simulink library "SolarCollector"  (R2018b)
settings: Solver=ode45  StartTime=0.0  StopTime=10.0  RelTol=1e-3  EnableMultiTasking=on
undefined symbols (not defined in the file): path_carnot
libraries: carnot x5
settings Model: Creator=bernd.hafner  LastModifiedBy=drhf
settings DataIOCC: LimitDataPoints=on  SaveFormat=Array  SignalLoggingSaveFormat=ModelDataLogs
settings OptimizationCC: ExpressionDepthLimit=2147483647  LifeSpan=inf
settings DebuggingCC: UnderspecifiedInitializationDetection=Classic  MergeDetectMultiDrivingBlocksExec=none  SolverPrmCheckMsg=warning  FcnCallInpInsideContextMsg=warning  StateNameClashWarn=warning  SFUnexpectedBacktrackingDiag=warning  SFNoUnconditionalDefaultTransitionDiag=warning  SFExecutionAtInitializationDiag=none
settings HardwareCC: ProdBitPerPointer=32  ProdBitPerSizeT=32  ProdBitPerPtrDiffT=32  ProdLargestAtomicFloat=None  ProdIntDivRoundTo=Undefined  ProdEndianess=Unspecified  ProdWordSize=32  ProdHWDeviceType=32-bit Generic
settings ModelReferenceCC: PropagateSignalLabelsOutOfModel=off
settings SFSimCC: SimUseLocalCustomCode=off
settings RTWCC: RTWUseLocalCustomCode=off
settings CodeAppCC: StateflowObjectComments=on
settings GRTTargetCC: TargetLangStandard=C89/C90 (ANSI)  GeneratePreprocessorConditionals=Disable all  CombineOutputUpdateFcns=off  GRTInterface=on
settings ConfigComp: CovMetricSettings=dw  CovHtmlReporting=on  CovSaveCumulativeToWorkspaceVar=on  CovSaveSingleToWorkspaceVar=on  CovExternalEMLEnable=off

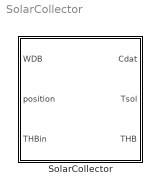
== system SolarCollector ==
  SolarCollector : Subsystem  mask(Solar Thermal Collector){t0=20, Ncollector=1, PathName=fullfile(path_carnot('libsl'), 'Source', 'Solar_Thermal', 'SolarCollector', 'parameter_set'), FileName='DefaultCollector.mat', userPath=off, userParam=off, acol=3.5, len=0.1, fta=0.7, c1=1.1, c2=0.001, c3=0, c4=0, c5=5000, c6=0, KbAngles=[0 5 10 15 20 25 30 35 40 45 50 55 60 65 70 75 80 85 90], KbL=[1 1 0.9999 0.9996 0.9991 0.9982 0.9965 0.9935 0.9886 0.9807 0.9678 0.9473 0.9148 0.8638 0.7846 0.6644 0.4907 0.2599 0], KbT=[1 1 1 1 1 1 1 1 1 1 1 0.875 0.75 0.625 0.5 0.375 0.25 0.125 0], Kd=0.92, dplin=10, dpqua=10, SensorTimeConstant=10}
      mask prompts: t0 "Initial temperature [°C]"; Ncollector "Number of collectors in parallel"; PathName "Path"; FileName "Parameter set"; userPath "Edit path and name of parameter set"; userParam "User defined parameters"; acol "A: surface  of one collector module in m²"; len "Length between collector inlet and outlet in m"; fta "Fin Efficiency * Transmission * Absorption (F'(tau alfa))"; c1 "c1 : heat loss coefficient at (Tm-Ta)=0  [W/(m²*K)]"; c2 "c2: temperature dependence of the heat loss coefficient [W/(m*K)²]"; c3 "c3 : wind speed dependence of the heat loss coefficient [J/(m³K)]"; c4 "c4 : sky temperature dependence of the heat loss coefficient [W/(m²K)]"; c5 "c5 : effective thermal capacity [J/(m²K)]"; c6 "c6 : wind dependence in the zero loss efficiency [s/m]"; KbAngles "Kb: angles for longitudinal and transversal IAM [degree]"; KbL "KbL: values for longitudinal incidence angle modifier (0..1)"; KbT "KbT: values for transversal incidence angle modifier (0..1)"; Kd "Kd : Incidence angle modifier diffuse radiation"; dplin "lin: linear pressure drop in Pa/(kg/s)"; dpqua "qua: quadratic pressure drop in Pa/(kg/s)²"; SensorTimeConstant "time constant of sensor [s]"
      mask help:
      | Model for glazed solar thermal collector according to ISO 9806 standard.
      | c5 dTm/dt = F'(TauAlfa) (Kdir Idir + Kdfu Idfu) - (Tm-Tamb) (c1 + c2 (Tm-Tamb)) - v_wind (c3 (Tm-Ta) + c6 Iglb) + c4 (ELongwave - sigma_SB Tamb^4) - mdot cp (Tout-Tin) /A
      | Tm = (Tin+Tout)/2
      | Keep in mind that the ISO equation is not respecting the energy conservation for variable inlet conditions (e.g. temperature).
      | IT IS RECOMMENDED TO USE THIS MODEL ONLY FOR STEADY STATE CONDITIONS AT THE INLET (use Collector_Unglazed_ISO_2node model for system simulation).
      mask init:
      | % callback to set parameters of model
      | [ok, param] = CarnotCallbacks_CollectorEN12975Conf('SetParameters',gcbh,PathName,FileName);
      mask Help: web(fullfile(path_carnot('help'),'collector_en12975.html'),'-helpbrowser')
      mask TypeOptions t0: T_Sensor/t0 | glazed_collector_ISO9806/tini
      mask TypeOptions Ncollector: Ncollector/Value | Gain1/Gain | Gain2/Gain
      mask Callback userPath: [ok, param] = CarnotCallbacks_CollectorEN12975Conf('UserEdit',gcbh);
      mask Callback userParam: [ok, param] = CarnotCallbacks_CollectorEN12975Conf('UserEdit',gcbh);
      mask TypeOptions acol: glazed_collector_ISO9806/acol | Acol/Value
      mask TypeOptions len: Pressure_Drop_Collector/len
      mask TypeOptions fta: glazed_collector_ISO9806/fta
      mask TypeOptions c1: glazed_collector_ISO9806/c1
      mask TypeOptions c2: glazed_collector_ISO9806/c2
      mask TypeOptions c3: glazed_collector_ISO9806/c3
      mask TypeOptions c4: glazed_collector_ISO9806/c4
      mask TypeOptions c5: glazed_collector_ISO9806/c5
      mask TypeOptions c6: glazed_collector_ISO9806/c6
      mask TypeOptions KbAngles: glazed_collector_ISO9806/kblangle | glazed_collector_ISO9806/kbtangle
      mask TypeOptions KbL: glazed_collector_ISO9806/KbL
      mask TypeOptions KbT: glazed_collector_ISO9806/KbT
      mask TypeOptions Kd: glazed_collector_ISO9806/Kd
      mask TypeOptions dplin: Pressure_Drop_Collector/lin
      mask TypeOptions dpqua: Pressure_Drop_Collector/qua
      mask TypeOptions SensorTimeConstant: T_Sensor/tc
      mask DialogControl ParameterGroupVar Prompt: Picking a parameter set
      mask DialogControl Control2 Prompt: Carnot public data
      mask DialogControl Control2 Callback: [ok, file] = CarnotCallbacks_CollectorEN12975Conf('GetFilename',gcbh,'public');
      mask DialogControl Control3 Prompt: Carnot internal data
      mask DialogControl Control3 Callback: [ok, file] = CarnotCallbacks_CollectorEN12975Conf('GetFilename',gcbh,'internal');
      mask DialogControl Control4 Prompt: Selected path
      mask DialogControl Control4 Callback: [ok, file] = CarnotCallbacks_CollectorEN12975Conf('GetFilename',gcbh,'selected');
      mask DialogControl Container7 Prompt: Geometry
      mask DialogControl Container8 Prompt: Coll.Params
      mask DialogControl Container9 Prompt: Optics
      mask DialogControl Container10 Prompt: Hydraulic
      mask DialogControl Container11 Prompt: Sensors
      mask DialogControl Control5 Prompt: Save in Carnot interal data
      mask DialogControl Control5 Callback: [ok, param] = CarnotCallbacks_CollectorEN12975Conf('SaveFilename',gcbh,'internal','COL');
      mask DialogControl Control6 Prompt: Save in seleced path
      mask DialogControl Control6 Callback: [ok, param] = CarnotCallbacks_CollectorEN12975Conf('SaveFilename',gcbh,'selected','COL');
      mask Display:
      | % user defined picture file
      | picfile = fullfile(path_carnot('intlibsl'), ...
      |     'Source','Solar_Thermal','SolarCollector','parameter_set', ...
      |      'Collector_CONF.jpg');
      | 
      | pic = false;
      | 
      | % show internal picture if defined
      | if ~BlockIsInCarnotLibrary    % if not located in library any more
      |     if exist(picfile)
      |         image(imread(picfile), [0.2, 0, 0.6, 1])
      |         set_param(gcb, 'BackgroundColor', 'White')
      |         pic = true;
      |     end
      | end
      | 
      | if ~pic    % show public picture
      |     disp('Solar Thermal\nCollector\n\nISO 9806')
      |     set_param(gcb, 'BackgroundColor', 'Yellow')
      | end

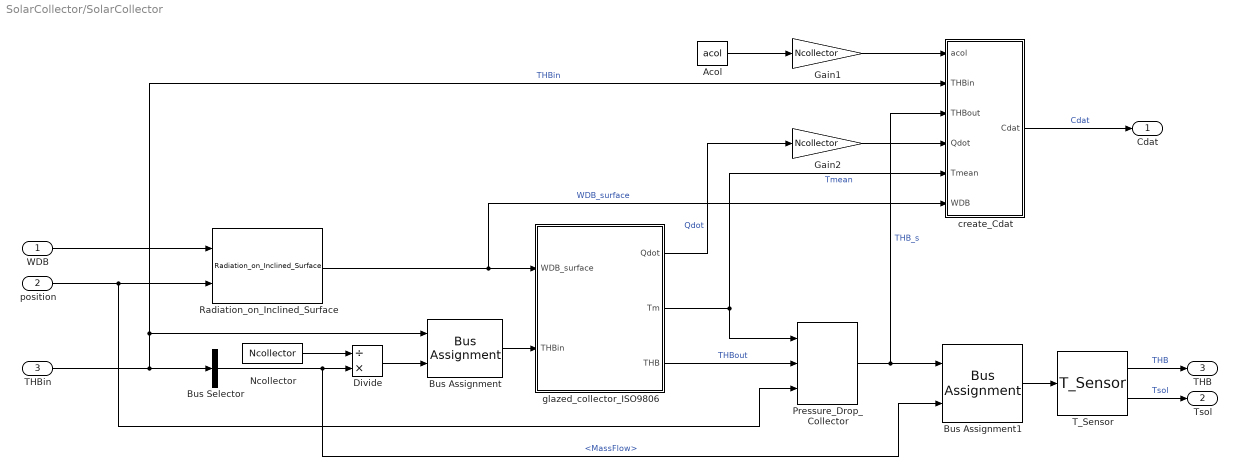
== system SolarCollector/SolarCollector ==
  WDB : Inport
  position : Inport  Port=2
  THBin : Inport  Port=3
  Acol : Constant  Value=acol
  Bus Assignment : BusAssignment  AssignedSignals=MassFlow
  Bus Assignment1 : BusAssignment  AssignedSignals=MassFlow
  Bus Selector : BusSelector  OutputSignals=MassFlow
  Divide : Product  Inputs=/*
  Gain1 : Gain  Gain=Ncollector
  Gain2 : Gain  Gain=Ncollector
  Ncollector : Constant  Value=Ncollector
  Pressure_Drop_Collector : carnot/Basic/Pressure_Drop/Pressure_Drop_Collector  len=len  lin=dplin  qua=dpqua
      settings: SourceProductName=Carnot
  Radiation_on_Inclined_Surface : carnot/Weather/Radiation_on_Inclined_Surface  sky=Perez 1990  reflect=0.2
      settings: SourceProductName=Carnot
  T_Sensor : carnot/Control/T_Sensor  tc=SensorTimeConstant  t0=t0
      settings: SourceProductName=Carnot
  create_Cdat : Subsystem
  glazed_collector_ISO9806 : Subsystem  mask(Basic Solar Thermal Collector){acol=acol, fta=fta, c1=c1, c2=c2, c3=c3, c4=c4, c5=c5, c6=c6, tini=t0, kblangle=KbAngles, KbL=KbL, kbtangle=KbAngles, KbT=KbT, Kd=Kd}
      mask prompts: acol "A : collector surface  [m²]"; fta "Fin Efficiency * Transmission * Absorption (F'(tau alfa))"; c1 "c1 : heat loss coefficient at (Tm-Ta)=0  [W/(m²*K)]"; c2 "c2: temperature dependence of the heat loss coefficient [W/(m*K)²]"; c3 "c3 : wind speed dependence of the heat loss coefficient [J/(m³K)]"; c4 "c4 : sky temperature dependence of the heat loss coefficient [W/(m²K)]"; c5 "c5 : effective thermal capacity [J/(m²K)]"; c6 "c6 : wind dependence in the zero loss efficiency [s/m]"; tini "initial temperature [degree Celsius]"; kblangle "KbL: angles for longitudinal IAM [degree]"; KbL "KbL: values for longitudinal incidence angle modifier (0..1)"; kbtangle "KbT: angles for transversal IAM [degree]"; KbT "KbT: values for transversal incidence angle modifier (0..1)"; Kd "Kd : Incidence angle modifier diffuse radiation"
      mask help: Model according to EN 12975 / ISO 22975
      mask Help: web(fullfile(path_carnot('help'),'Solar_Collector_basic.html'),'-helpbrowser')
      mask TypeOptions fta: IAM_Table_KbL_KbT/fta
      mask TypeOptions kblangle: IAM_Table_KbL_KbT/kblangle
      mask TypeOptions KbL: IAM_Table_KbL_KbT/KbL
      mask TypeOptions kbtangle: IAM_Table_KbL_KbT/kbtangle
      mask TypeOptions KbT: IAM_Table_KbL_KbT/KbT
      mask TypeOptions Kd: IAM_Table_KbL_KbT/Kd
      mask DialogControl Container4 Prompt: Collector Parameters
      mask DialogControl Container10 Prompt: Optics
      mask Display: disp('glazed\nsolar\nthermal\ncollector\nISO 9806')
  Cdat : Outport
  Tsol : Outport  Port=2
  THB : Outport  Port=3
  wires:
  Bus Assignment/1 -> glazed_collector_ISO9806/2(THBin)
  T_Sensor/1 -> THB/1  "THB"
  T_Sensor/2 -> Tsol/1  "Tsol"
  Divide/1 -> Bus Assignment/2
  Ncollector/1 -> Divide/1
  WDB/1 -> Radiation_on_Inclined_Surface/1
  glazed_collector_ISO9806/1(Qdot) -> Gain2/1  "Qdot"
  glazed_collector_ISO9806/3(THB) -> Pressure_Drop_Collector/2  "THBout"
  THBin/1 -> Bus Selector/1, create_Cdat/2(THBin), Bus Assignment/1  "THBin"
  glazed_collector_ISO9806/2(Tm) -> Pressure_Drop_Collector/1, create_Cdat/5(Tmean)  "Tmean"
  create_Cdat/1(Cdat) -> Cdat/1  "Cdat"
  Radiation_on_Inclined_Surface/1 -> glazed_collector_ISO9806/1(WDB_surface), create_Cdat/6(WDB)  "WDB_surface"
  Pressure_Drop_Collector/1 -> create_Cdat/3(THBout), Bus Assignment1/1  "THB_s"
  position/1 -> Pressure_Drop_Collector/3, Radiation_on_Inclined_Surface/2
  Acol/1 -> Gain1/1
  Bus Selector/1 -> Bus Assignment1/2, Divide/2  "<MassFlow>"
  Gain1/1 -> create_Cdat/1(acol)
  Gain2/1 -> create_Cdat/4(Qdot)
  Bus Assignment1/1 -> T_Sensor/1

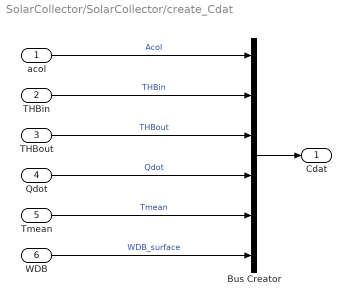
== system SolarCollector/SolarCollector/create_Cdat ==
  acol : Inport
  THBin : Inport  Port=2
  THBout : Inport  Port=3
  Qdot : Inport  Port=4
  Tmean : Inport  Port=5
  WDB : Inport  Port=6
  Bus Creator : BusCreator  Inputs=6
  Cdat : Outport
  wires:
  Tmean/1 -> Bus Creator/5  "Tmean"
  Qdot/1 -> Bus Creator/4  "Qdot"
  Bus Creator/1 -> Cdat/1
  WDB/1 -> Bus Creator/6  "WDB_surface"
  THBout/1 -> Bus Creator/3  "THBout"
  THBin/1 -> Bus Creator/2  "THBin"
  acol/1 -> Bus Creator/1  "Acol"

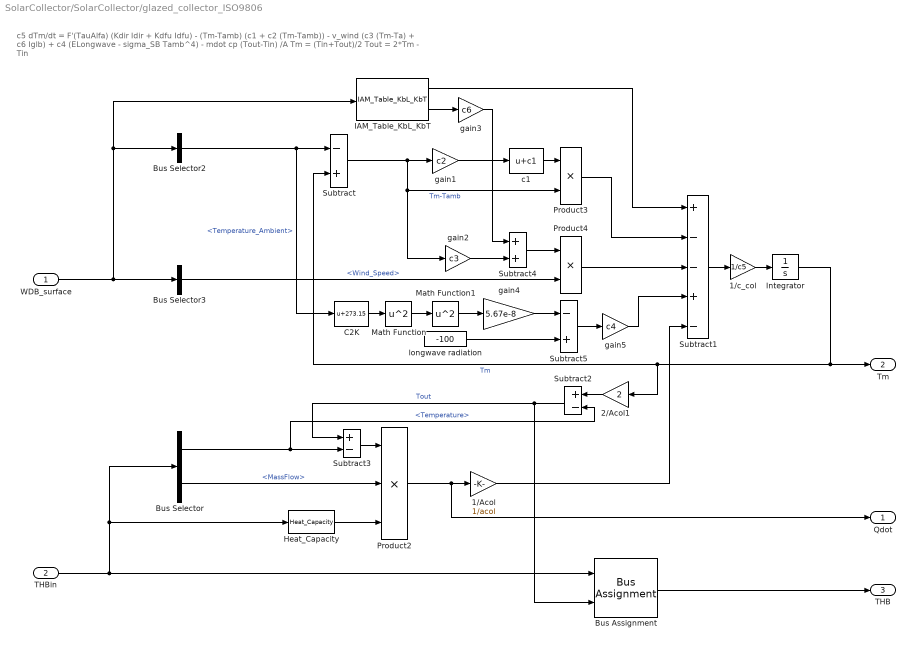
== system SolarCollector/SolarCollector/glazed_collector_ISO9806 ==
  note: c5 dTm/dt = F'(TauAlfa) (Kdir Idir + Kdfu Idfu) - (Tm-Tamb) (c1 + c2 (Tm-Tamb)) - v_wind (c3 (Tm-Ta) + c6 Iglb) + c4 (ELongwave - sigma_SB Tamb^4) - mdot cp (Tout-Tin) /A
      | Tm = (Tin+Tout)/2
      | Tout = 2*Tm - Tin
  WDB_surface : Inport
  THBin : Inport  Port=2
  1/Acol : Gain  Gain=1/acol
  1/c_col : Gain  Gain=1/c5
  2/Acol1 : Gain  Gain=2
  Bus Assignment : BusAssignment  AssignedSignals=Temperature
  Bus Selector : BusSelector  OutputSignals=Temperature,MassFlow
  Bus Selector2 : BusSelector  OutputSignals=Temperature_Ambient
  Bus Selector3 : BusSelector  OutputSignals=Wind_Speed
  C2K : Bias  Bias=273.15
  Heat_Capacity : carnot/Basic/Material_Properties/Heat_Capacity  VariantControl=CarlibClassic  INPUTARGUMENTS=THB  DEBUGLEVEL=DEBUGLEVEL  MAXTOTALWARNINGS=inf  MAXCONSECUTIVEWARNINGS=inf  WRITETOFILE=0  FILENAME='errors.txt'
      settings: SourceProductName=Carnot
  IAM_Table_KbL_KbT : carnot/Source/Solar_Thermal/IncidenceAngleModifier/IAM_Table_KbL_KbT  fta=fta  kblangle=kblangle  KbL=KbL  kbtangle=kbtangle  KbT=KbT  Kd=Kd
      settings: SourceProductName=Carnot
  Integrator : Integrator  InitialCondition=tini
  Math Function : Math  Operator=square  SaturateOnIntegerOverflow=on
  Math Function1 : Math  Operator=square  SaturateOnIntegerOverflow=on
  Product2 : Product  Inputs=3  RndMeth=Zero
  Product3 : Product  RndMeth=Zero
  Product4 : Product  RndMeth=Zero
  Subtract : Sum  Inputs=-+
  Subtract1 : Sum  Inputs=+--+-
  Subtract2 : Sum  Inputs=+-
  Subtract3 : Sum  Inputs=+-
  Subtract4 : Sum  Inputs=2
  Subtract5 : Sum  Inputs=-+
  c1 : Bias  Bias=c1
  gain1 : Gain  Gain=c2
  gain2 : Gain  Gain=c3
  gain3 : Gain  Gain=c6
  gain4 : Gain  Gain=5.67e-8
  gain5 : Gain  Gain=c4
  longwave radiation : Constant  Value=-100
  Qdot : Outport  InitialOutput=0
  Tm : Outport  Port=2  InitialOutput=0
  THB : Outport  Port=3  InitialOutput=0
  wires:
  Bus Assignment/1 -> THB/1
  Bus Selector/2 -> Product2/2  "<MassFlow>"
  Bus Selector/1 -> Subtract3/2, Subtract2/2  "<Temperature>"
  c1/1 -> Product3/1
  Subtract1/1 -> 1/c_col/1
  gain4/1 -> Subtract5/1
  gain3/1 -> Subtract4/1
  Subtract5/1 -> gain5/1
  Bus Selector3/1 -> Product4/2  "<Wind_Speed>"
  IAM_Table_KbL_KbT/1 -> Subtract1/1
  THBin/1 -> Bus Selector/1, Heat_Capacity/1, Bus Assignment/1
  Math Function1/1 -> gain4/1
  Product4/1 -> Subtract1/3
  1/c_col/1 -> Integrator/1
  Product3/1 -> Subtract1/2
  gain2/1 -> Subtract4/2
  gain1/1 -> c1/1
  Bus Selector2/1 -> Subtract/1, C2K/1  "<Temperature_Ambient>"
  Subtract3/1 -> Product2/1
  IAM_Table_KbL_KbT/2 -> gain3/1
  Product2/1 -> 1/Acol/1, Qdot/1
  Integrator/1 -> Subtract/2, 2/Acol1/1, Tm/1  "Tm"
  Heat_Capacity/1 -> Product2/3
  Subtract2/1 -> Subtract3/1, Bus Assignment/2  "Tout"
  1/Acol/1 -> Subtract1/5
  Subtract/1 -> gain2/1, Product3/2, gain1/1  "Tm-Tamb"
  2/Acol1/1 -> Subtract2/1
  Math Function/1 -> Math Function1/1
  gain5/1 -> Subtract1/4
  longwave radiation/1 -> Subtract5/2
  C2K/1 -> Math Function/1
  Subtract4/1 -> Product4/1
  WDB_surface/1 -> Bus Selector2/1, IAM_Table_KbL_KbT/1, Bus Selector3/1
